simulink model "windup3"  (R2021a)
settings: Solver=VariableStepAuto  StartTime=0.0  StopTime=Tmax  RelTol=1e-3
values from neighbouring files (symbols this model uses):
  Kd = 2.7    [windup2_test.m]
  N = numel(Gall)    [ultgain.m]    (also in windup2_test.m = 10; windup_test.m = 10)
  S = 0.1    [windup2_test.m]    (also in windup_test.m = 4)
  Td = 0.8    [windup2_test.m]    (also in windup_test.m = 1)
  Ti = 7.5    [windup2_test.m]    (also in windup_test.m = 1; workshop7.m = 1.6)
libraries: simulink x1
settings Model: Creator=will  LastModifiedBy=will
settings SolverCC: AlgebraicLoopSolver=TrustRegion
settings DataIOCC: ReturnWorkspaceOutputs=off
settings DebuggingCC: SFMachineParentedDataDiag=warning  ArithmeticOperatorsInVariantConditions=warning
settings SFSimCC: SimUseLocalCustomCode=off  CustomCodeUndefinedFunction=UseInterfaceOnly
settings RTWCC: RTWUseLocalCustomCode=off

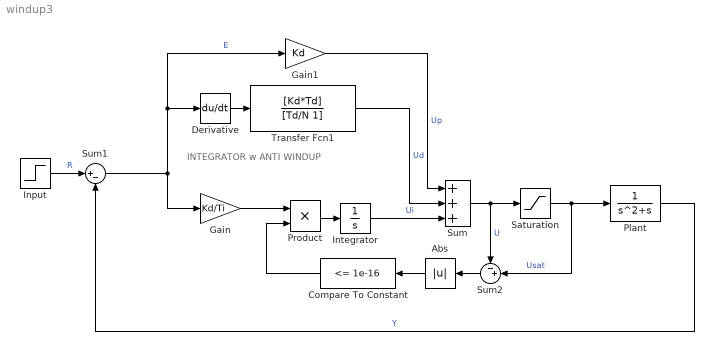
== system windup3 ==
  note: INTEGRATOR w ANTI WINDUP
  Abs : Abs
  Compare To Constant : simulink/Logic and Bit Operations/Compare To Constant  relop=<=  const=1e-16  OutDataTypeStr=boolean
  Derivative : Derivative
  Gain : Gain  Gain=Kd/Ti
  Gain1 : Gain  Gain=Kd
  Input : Step  SampleTime=0
  Integrator : Integrator
  Plant : TransferFcn  Denominator=[1 1 0]
  Product : Product
  Saturation : Saturate  UpperLimit=S  LowerLimit=-S
  Sum : Sum  Inputs=+++
  Sum1 : Sum  Inputs=|+-
  Sum2 : Sum  Inputs=-+|
  Transfer Fcn1 : TransferFcn  Numerator=[Kd*Td]  Denominator=[Td/N 1]
  wires:
  Gain1/1 -> Sum/1  "Up"
  Integrator/1 -> Sum/3  "Ui"
  Transfer Fcn1/1 -> Sum/2  "Ud"
  Sum1/1 -> Gain1/1, Derivative/1, Gain/1  "E"
  Sum/1 -> Sum2/1, Saturation/1  "U"
  Derivative/1 -> Transfer Fcn1/1
  Saturation/1 -> Plant/1, Sum2/2  "Usat"
  Plant/1 -> Sum1/2  "Y"
  Input/1 -> Sum1/1  "R"
  Gain/1 -> Product/1
  Product/1 -> Integrator/1
  Sum2/1 -> Abs/1
  Abs/1 -> Compare To Constant/1
  Compare To Constant/1 -> Product/2
